simulink model "controller_ap_cfb"  (R2020a)
settings: Solver=FixedStepDiscrete  StartTime=0.0  StopTime=10.0  FixedStep=0.001  MaxStep=0.01  RelTol=1e-3
libraries: simulink x2
settings Model: Creator=upattacini  LastModifiedBy=upattacini
settings SolverCC: MaxConsecutiveMinStep=10

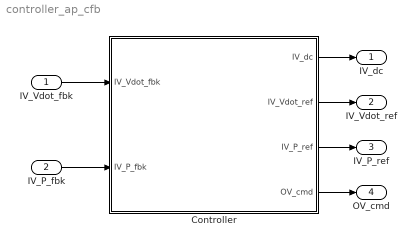
== system controller_ap_cfb ==
  IV_Vdot_fbk : Inport
  IV_P_fbk : Inport  Port=2
  Controller : Subsystem  Tag=PublishSubsystem  mask(Controller){Ts=0.001, control_mode=Volume Control, tidal_volume=0.65, PIP=25, PEEP=5, respiratory_rate=8, IE_ratio=1/3}
      mask prompts: Ts "Sample Time (s)"; control_mode "Control Mode"; tidal_volume "Tidal Volume (L)"; PIP "Peak Inspiratory Pressure (cmH20)"; PEEP "PEEP (cmH20)"; respiratory_rate "Respiratory Rate (breaths/min)"; IE_ratio "Inspiration to Expiration Ratio"
      mask help: The controller generates the input signals that controls the inspiratory flow and expiratory valve.
      mask init:
      | mode = get_param(gcb,'control_mode');
      | vc_mode = strcmpi(mode, 'Volume Control');
      | pc_mode = strcmpi(mode, 'Pressure Control');
      | 
      | pc_tau = (IE_ratio/(IE_ratio+1) * (60 / respiratory_rate)) * (2/3) / 4;
      mask TypeOptions control_mode: Volume Control | Pressure Control
      mask Callback control_mode:
      | mode = get_param(gcb,'control_mode');
      | if strcmpi(mode, 'Volume Control')
      |     set_param(gcb, 'MaskEnableString', 'on,on,on,off,off,on,on');
      | else
      |     set_param(gcb, 'MaskEnableString', 'on,on,off,on,on,on,on');
      | end
  IV_dc : Outport
  IV_Vdot_ref : Outport  Port=2
  IV_P_ref : Outport  Port=3
  OV_cmd : Outport  Port=4
  wires:
  IV_Vdot_fbk/1 -> Controller/1(IV_Vdot_fbk)
  Controller/1(IV_dc) -> IV_dc/1
  Controller/2(IV_Vdot_ref) -> IV_Vdot_ref/1
  Controller/4(OV_cmd) -> OV_cmd/1
  IV_P_fbk/1 -> Controller/2(IV_P_fbk)
  Controller/3(IV_P_ref) -> IV_P_ref/1

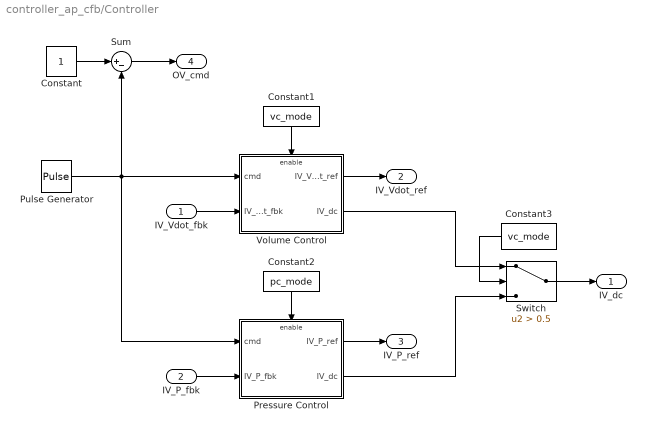
== system controller_ap_cfb/Controller ==
  IV_Vdot_fbk : Inport
  IV_P_fbk : Inport  Port=2
  Constant : Constant
  Constant1 : Constant  Value=vc_mode
  Constant2 : Constant  Value=pc_mode
  Constant3 : Constant  Value=vc_mode
  Pressure Control : Subsystem
  Pulse Generator : DiscretePulseGenerator  Period=floor((60 / respiratory_rate) / Ts)  PulseWidth=floor((IE_ratio/(IE_ratio+1) * (60 / respiratory_rate)) / Ts)  SampleTime=Ts
  Sum : Sum  Inputs=|+-
  Switch : Switch  Criteria=u2 > Threshold  Threshold=0.5
  Volume Control : Subsystem
  IV_dc : Outport
  IV_Vdot_ref : Outport  Port=2
  IV_P_ref : Outport  Port=3
  OV_cmd : Outport  Port=4
  wires:
  Pulse Generator/1 -> Pressure Control/1(cmd), Sum/2, Volume Control/1(cmd)
  Constant/1 -> Sum/1
  Sum/1 -> OV_cmd/1
  IV_Vdot_fbk/1 -> Volume Control/2(IV_Vdot_fbk)
  Volume Control/1(IV_Vdot_ref) -> IV_Vdot_ref/1
  Constant1/1 -> Volume Control/Enable
  Constant2/1 -> Pressure Control/Enable
  Switch/1 -> IV_dc/1
  Volume Control/2(IV_dc) -> Switch/1
  Pressure Control/2(IV_dc) -> Switch/3
  Constant3/1 -> Switch/2
  IV_P_fbk/1 -> Pressure Control/2(IV_P_fbk)
  Pressure Control/1(IV_P_ref) -> IV_P_ref/1

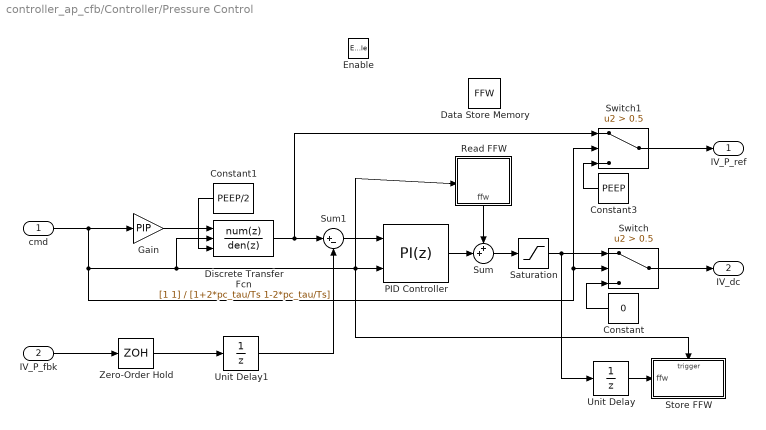
== system controller_ap_cfb/Controller/Pressure Control ==
  cmd : Inport
  IV_P_fbk : Inport  Port=2
  Enable : EnablePort
  Constant : Constant  Value=0
  Constant1 : Constant  Value=PEEP/2
  Constant3 : Constant  Value=PEEP
  Data Store Memory : DataStoreMemory  DataStoreName=FFW  ReadBeforeWriteMsg=warning  WriteAfterWriteMsg=warning  WriteAfterReadMsg=warning  ShowAdditionalParam=off  OutMin=0  OutMax=100
  Discrete Transfer Fcn : DiscreteTransferFcn  Numerator=[1 1]  Denominator=[1+2*pc_tau/Ts 1-2*pc_tau/Ts]  InitialStatesSource=Input port  InitialStates=PEEP  ExternalReset=Rising
      settings: InputPortMap=u0,r7,p5
  Gain : Gain  Gain=PIP
  PID Controller : simulink/Continuous/PID Controller  Controller=PI  Form=Parallel  TimeDomain=Discrete-time  UseExternalTs=off  SampleTime=-1  IntegratorMethod=Trapezoidal  FilterMethod=Trapezoidal  ControllerParametersSource=internal  P=15  I=30  D=1  UseFilter=on  N=100  TunerSelectOption=Transfer Function Based (PID Tuner App)  InitialConditionSource=internal  InitialConditionForIntegrator=0  InitialConditionForFilter=0  DifferentiatorICPrevScaledInput=0  ExternalReset=rising  TrackingMode=off  Kt=1  LimitOutput=off  UpperSaturationLimit=100  LowerSaturationLimit=0  LinearizeAsGain=on  AntiWindupMode=clamping  Kb=1  POutMin=[]  POutMax=[]  IOutMin=[]  IOutMax=[]  DOutMin=[]  DOutMax=[]  NOutMin=[]  NOutMax=[]  SumOutMin=[]  SumOutMax=[]  SaturationOutMin=[]  SaturationOutMax=[]  PParamMin=[]  PParamMax=[]  IParamMin=[]  IParamMax=[]  DParamMin=[]  DParamMax=[]  NParamMin=[]  NParamMax=[]  KbParamMin=[]  KbParamMax=[]  KtParamMin=[]  KtParamMax=[]  KbOutMin=[]  KbOutMax=[]  KtOutMin=[]  KtOutMax=[]  IntegratorOutMin=[]  IntegratorOutMax=[]  FilterOutMin=[]  FilterOutMax=[]  SumI1OutMin=[]  SumI1OutMax=[]  SumI2OutMin=[]  SumI2OutMax=[]  SumI3OutMin=[]  SumI3OutMax=[]  SumI4OutMin=[]  SumI4OutMax=[]  SumDOutMin=[]  SumDOutMax=[]  DifferentiatorOutMin=[]  DifferentiatorOutMax=[]  FilterDiffOutCoefMin=[]  FilterDiffOutCoefMax=[]  ReciprocalOutMin=[]  ReciprocalOutMax=[]  SumDenOutMin=[]  SumDenOutMax=[]  SumNumOutMin=[]  SumNumOutMax=[]  DivideOutMin=[]  DivideOutMax=[]  UdiffTsProdOutMin=[]  UdiffTsProdOutMax=[]  NTsProdOutMin=[]  NTsProdOutMax=[]  UintegralTsProdOutMin=[]  UintegralTsProdOutMax=[]  UngainTsProdOutMin=[]  UngainTsProdOutMax=[]  IntegratorContinuousStateAttributes=''  IntegratorStateMustResolveToSignalObject=off  IntegratorRTWStateStorageClass=Auto  FilterContinuousStateAttributes=''  FilterStateMustResolveToSignalObject=off  FilterRTWStateStorageClass=Auto  ParallelPVariant=InternalParameters  IdealPVariant=Disabled  IVariant=InternalParameters  DVariant=Disabled  IntegratorVariant=Discrete  SatVariant=Disabled  AWVariant=Passthrough  PCopyVariant=Disabled  TRVariant=Disabled  FdbkBlocksVariant=Forward  IdealPFdbkVariant=Disabled  SatFdbkVariant=Disabled  DerivativeFilterVariant=Disabled  NVariant=Disabled  NCopyVariant=Disabled_SignalSpec  FilterICVariant=Disabled  IntegratorICVariant=InternalICs  ExternalResetVariant=ExternalReset  TRSumVariant=Passthrough  SumFdbkVariant=Disabled  SumVariant=Sum_PI  TsampFilterVariant=InternalTs  TsampNgainVariant=Passthrough  TsampIntegralVariant=Passthrough
  Read FFW : Subsystem  TreatAsAtomicUnit=on
  Saturation : Saturate  UpperLimit=100  LowerLimit=0
  Store FFW : Subsystem  TreatAsAtomicUnit=on
  Sum : Sum  Inputs=++|
  Sum1 : Sum  Inputs=|+-
  Switch : Switch  Criteria=u2 > Threshold  Threshold=0.5
  Switch1 : Switch  Criteria=u2 > Threshold  Threshold=0.5
  Unit Delay : UnitDelay  SampleTime=-1  HasFrameUpgradeWarning=on
  Unit Delay1 : UnitDelay  SampleTime=-1  HasFrameUpgradeWarning=on
  Zero-Order Hold : ZeroOrderHold  SampleTime=Ts
  IV_P_ref : Outport
  IV_dc : Outport  Port=2
  wires:
  IV_P_fbk/1 -> Zero-Order Hold/1
  Unit Delay1/1 -> Sum1/2
  Sum1/1 -> PID Controller/1
  cmd/1 -> Switch1/2, Switch/2, Store FFW/Trigger, Read FFW/Enable, PID Controller/2, Discrete Transfer Fcn/2, Gain/1
  Zero-Order Hold/1 -> Unit Delay1/1
  Discrete Transfer Fcn/1 -> Sum1/1, Switch1/1
  Saturation/1 -> Unit Delay/1, Switch/1
  Switch/1 -> IV_dc/1
  Constant/1 -> Switch/3
  Switch1/1 -> IV_P_ref/1
  Gain/1 -> Discrete Transfer Fcn/1
  PID Controller/1 -> Sum/2
  Sum/1 -> Saturation/1
  Read FFW/1(ffw) -> Sum/1
  Constant1/1 -> Discrete Transfer Fcn/3
  Constant3/1 -> Switch1/3
  Unit Delay/1 -> Store FFW/1(ffw)

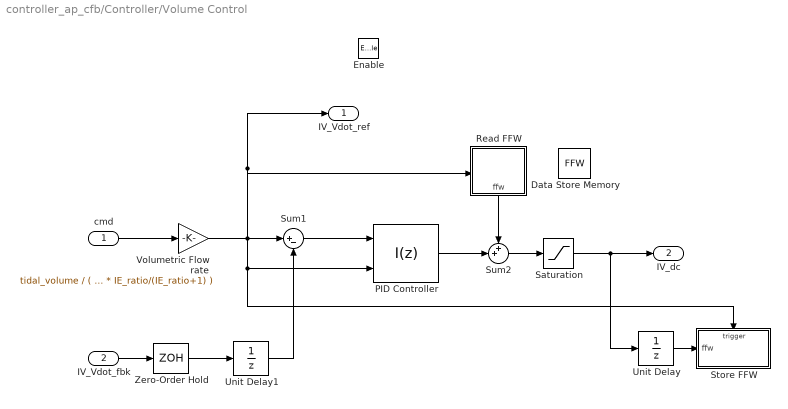
== system controller_ap_cfb/Controller/Volume Control ==
  cmd : Inport
  IV_Vdot_fbk : Inport  Port=2
  Enable : EnablePort
  Data Store Memory : DataStoreMemory  DataStoreName=FFW  ReadBeforeWriteMsg=warning  WriteAfterWriteMsg=warning  WriteAfterReadMsg=warning  ShowAdditionalParam=off  OutMin=0  OutMax=100
  PID Controller : simulink/Continuous/PID Controller  Controller=I  Form=Parallel  TimeDomain=Discrete-time  UseExternalTs=off  SampleTime=-1  IntegratorMethod=Trapezoidal  FilterMethod=Forward Euler  ControllerParametersSource=internal  P=0.5  I=10  D=1  UseFilter=on  N=100  TunerSelectOption=Transfer Function Based (PID Tuner App)  InitialConditionSource=internal  InitialConditionForIntegrator=0  InitialConditionForFilter=0  DifferentiatorICPrevScaledInput=0  ExternalReset=falling  TrackingMode=off  Kt=1  LimitOutput=off  UpperSaturationLimit=100  LowerSaturationLimit=0  LinearizeAsGain=on  AntiWindupMode=clamping  Kb=1  POutMin=[]  POutMax=[]  IOutMin=[]  IOutMax=[]  DOutMin=[]  DOutMax=[]  NOutMin=[]  NOutMax=[]  SumOutMin=[]  SumOutMax=[]  SaturationOutMin=[]  SaturationOutMax=[]  PParamMin=[]  PParamMax=[]  IParamMin=[]  IParamMax=[]  DParamMin=[]  DParamMax=[]  NParamMin=[]  NParamMax=[]  KbParamMin=[]  KbParamMax=[]  KtParamMin=[]  KtParamMax=[]  KbOutMin=[]  KbOutMax=[]  KtOutMin=[]  KtOutMax=[]  IntegratorOutMin=[]  IntegratorOutMax=[]  FilterOutMin=[]  FilterOutMax=[]  SumI1OutMin=[]  SumI1OutMax=[]  SumI2OutMin=[]  SumI2OutMax=[]  SumI3OutMin=[]  SumI3OutMax=[]  SumI4OutMin=[]  SumI4OutMax=[]  SumDOutMin=[]  SumDOutMax=[]  DifferentiatorOutMin=[]  DifferentiatorOutMax=[]  FilterDiffOutCoefMin=[]  FilterDiffOutCoefMax=[]  ReciprocalOutMin=[]  ReciprocalOutMax=[]  SumDenOutMin=[]  SumDenOutMax=[]  SumNumOutMin=[]  SumNumOutMax=[]  DivideOutMin=[]  DivideOutMax=[]  UdiffTsProdOutMin=[]  UdiffTsProdOutMax=[]  NTsProdOutMin=[]  NTsProdOutMax=[]  UintegralTsProdOutMin=[]  UintegralTsProdOutMax=[]  UngainTsProdOutMin=[]  UngainTsProdOutMax=[]  IntegratorContinuousStateAttributes=''  IntegratorStateMustResolveToSignalObject=off  IntegratorRTWStateStorageClass=Auto  FilterContinuousStateAttributes=''  FilterStateMustResolveToSignalObject=off  FilterRTWStateStorageClass=Auto  ParallelPVariant=Disabled  IdealPVariant=Disabled  IVariant=InternalParameters  DVariant=Disabled  IntegratorVariant=Discrete  SatVariant=Disabled  AWVariant=Passthrough  PCopyVariant=Disabled  TRVariant=Disabled  FdbkBlocksVariant=Forward  IdealPFdbkVariant=Disabled  SatFdbkVariant=Disabled  DerivativeFilterVariant=Disabled  NVariant=Disabled  NCopyVariant=Disabled_SignalSpec  FilterICVariant=Disabled  IntegratorICVariant=InternalICs  ExternalResetVariant=ExternalReset  TRSumVariant=Passthrough  SumFdbkVariant=Disabled  SumVariant=Passthrough_I  TsampFilterVariant=InternalTs  TsampNgainVariant=Passthrough  TsampIntegralVariant=Passthrough
  Read FFW : Subsystem  TreatAsAtomicUnit=on
  Saturation : Saturate  UpperLimit=100  LowerLimit=0
  Store FFW : Subsystem  TreatAsAtomicUnit=on
  Sum1 : Sum  Inputs=|+-
  Sum2 : Sum  Inputs=++|
  Unit Delay : UnitDelay  SampleTime=-1  HasFrameUpgradeWarning=on
  Unit Delay1 : UnitDelay  SampleTime=-1  HasFrameUpgradeWarning=on
  Volumetric Flow rate : Gain  Gain=tidal_volume / ( (1/respiratory_rate) * IE_ratio/(IE_ratio+1) )
  Zero-Order Hold : ZeroOrderHold  SampleTime=Ts
  IV_Vdot_ref : Outport
  IV_dc : Outport  Port=2
  wires:
  Zero-Order Hold/1 -> Unit Delay1/1
  Read FFW/1(ffw) -> Sum2/1
  Volumetric Flow rate/1 -> PID Controller/2, Store FFW/Trigger, Sum1/1, IV_Vdot_ref/1, Read FFW/Enable
  cmd/1 -> Volumetric Flow rate/1
  Sum2/1 -> Saturation/1
  Saturation/1 -> IV_dc/1, Unit Delay/1
  Sum1/1 -> PID Controller/1
  PID Controller/1 -> Sum2/2
  Unit Delay/1 -> Store FFW/1(ffw)
  Unit Delay1/1 -> Sum1/2
  IV_Vdot_fbk/1 -> Zero-Order Hold/1

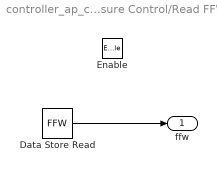
== system controller_ap_cfb/Controller/Pressure Control/Read FFW ==
  Enable : EnablePort
  Data Store Read : DataStoreRead  DataStoreName=FFW
  ffw : Outport  OutputWhenDisabled=reset  InitialOutput=0
  wires:
  Data Store Read/1 -> ffw/1

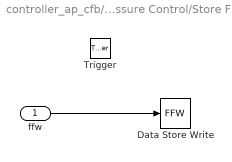
== system controller_ap_cfb/Controller/Pressure Control/Store FFW ==
  ffw : Inport
  Trigger : TriggerPort  TriggerType=falling  VariantControl=Variant  PortDimensions=1
  Data Store Write : DataStoreWrite  DataStoreName=FFW
  wires:
  ffw/1 -> Data Store Write/1

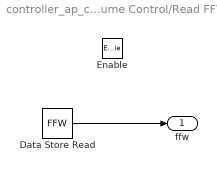
== system controller_ap_cfb/Controller/Volume Control/Read FFW ==
  Enable : EnablePort
  Data Store Read : DataStoreRead  DataStoreName=FFW
  ffw : Outport  OutputWhenDisabled=reset  InitialOutput=0
  wires:
  Data Store Read/1 -> ffw/1

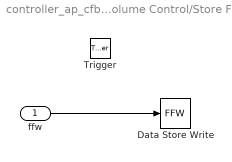
== system controller_ap_cfb/Controller/Volume Control/Store FFW ==
  ffw : Inport
  Trigger : TriggerPort  TriggerType=falling  VariantControl=Variant  PortDimensions=1
  Data Store Write : DataStoreWrite  DataStoreName=FFW
  wires:
  ffw/1 -> Data Store Write/1
